simulink model "RobotCode_R2022b"  (R2022b)
settings: Solver=ode3  StartTime=0.0  StopTime=inf  RelTol=1e-3  EnableMultiTasking=on
undefined symbols (not defined in the file or in its folder): CPR, DRV_GAIN, GR, T
libraries: cstblocks x8, simulink x8, arduinosensorlib x5, dspsigops x1
settings Model: FPTRunName=Active  ExtModeTrigDuration=2  Creator=20181889  LastModifiedBy=Rafael
settings SolverCC: AlgebraicLoopSolver=TrustRegion  AutoInsertRateTranBlk=on
settings DataIOCC: LimitDataPoints=on  SaveFormat=Array
settings OptimizationCC: ReuseModelBlockBuffer=on  ExpressionDepthLimit=2147483647  LifeSpan=Inf  MaxStackSize=64
settings DebuggingCC: UnderspecifiedInitializationDetection=Classic  MergeDetectMultiDrivingBlocksExec=none  FcnCallInpInsideContextMsg=warning  UnconnectedInputMsg=warning  UnconnectedOutputMsg=warning  UnconnectedLineMsg=warning  AllowSymbolicDim=off  StateNameClashWarn=warning  SFUnexpectedBacktrackingDiag=warning  SFNoUnconditionalDefaultTransitionDiag=warning  SFExecutionAtInitializationDiag=none  ArithmeticOperatorsInVariantConditions=warning
settings HardwareCC: ProdBitPerPointer=32  ProdBitPerSizeT=32  ProdBitPerPtrDiffT=32  ProdLargestAtomicInteger=Long  ProdLargestAtomicFloat=Double  ProdWordSize=32  ProdHWDeviceType=ARM Compatible->ARM Cortex
settings ModelReferenceCC: EnableRefExpFcnMdlSchedulingChecks=on  PropagateSignalLabelsOutOfModel=off
settings SFSimCC: SimUseLocalCustomCode=off  CustomCodeUndefinedFunction=UseInterfaceOnly
settings RTWCC: Description=Embedded Coder  SystemTargetFile=ert.tlc  HardwareBoard=Arduino Due  TemplateMakefile=ert_default_tmf  GenerateReport=on  RTWVerbose=off  RTWUseLocalCustomCode=off  Toolchain=Arduino ARM  BuildConfiguration=Faster Runs  LaunchReport=on
settings CodeAppCC: ForceParamTrailComments=on  OperatorAnnotations=on  StateflowObjectComments=on  MATLABSourceComments=on
settings ERTTargetCC: TargetLangStandard=C99 (ISO)  MultiwordLength=2048  ERTCustomFileBanners=off  SupportContinuousTime=on  SupportNonInlinedSFcns=on  RemoveResetFunc=off  SupportVariableSizeSignals=on  ModelStepFunctionPrototypeControlCompliant=off  ExtModeTransport=3  ExtModeStaticAlloc=on  ExtModeStaticAllocSize=24576  ExtModeMexFile=ext_xcp  ExtModeIntrfLevel=Level2 - Open
settings ConfigComp: CovMetricSettings=dw  CovSaveCumulativeToWorkspaceVar=on  CovSaveSingleToWorkspaceVar=on  CovExternalEMLEnable=off  CovSFcnEnable=off

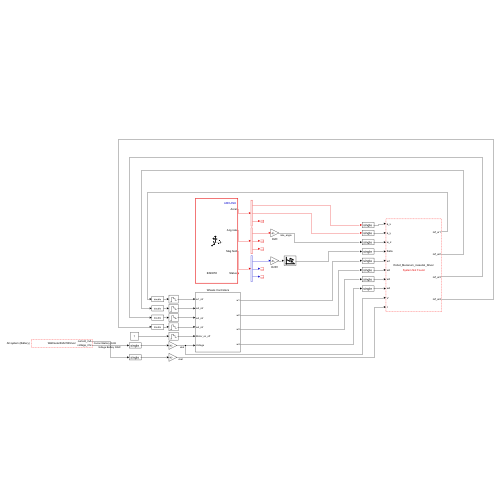
[thumbnail: Simulink's stored preview of the top-level diagram]
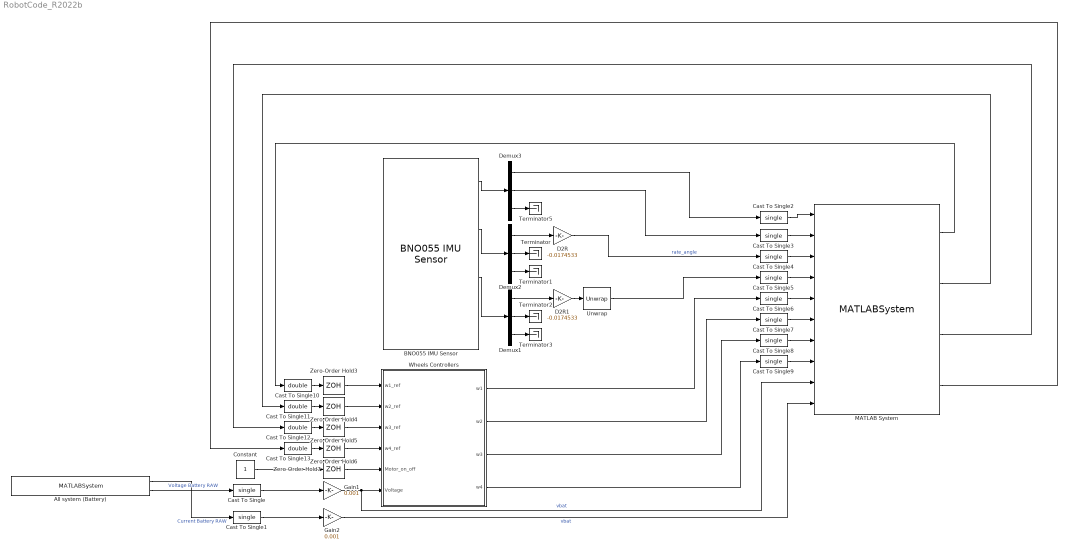
== system RobotCode_R2022b ==
  All system (Battery) : MATLABSystem  System=WattmeterINA219Driver  id=0  wire_number=0  address=45  SampleTime=T
      mask Type: WattmeterINA219Driver
      mask Display:
      | disp('WattmeterINA219Driver');
      | port_label('output',1,'current_mA');
      | port_label('output',2,'voltage_mV');
  BNO055 IMU Sensor : arduinosensorlib/BNO055 IMU Sensor  SlaveAddress=0x29  OperationMode=Fusion  Accel=on  AngularRate=on  MagField=off  EulerAngles=on  Quat=off  LinearAccel=off  GravityVector=off  Status=off  Timestamp=off  AccelRange=4G  AccelBW=62.5 Hz  GyroRange=2000 dps  GyroBW=32 Hz  MagODR=10 Hz  spf=1  SampleTime=T  blockPlatform=ARDUINO  QueueSizeFactor=1
  Cast To Single{,1..9} (10 alike) : DataTypeConversion  OutDataTypeStr=single  SaturateOnIntegerOverflow=off  RndMeth=Floor
  Cast To Single{10..13} (4 alike) : DataTypeConversion  OutDataTypeStr=double  SaturateOnIntegerOverflow=off  RndMeth=Floor
  Constant : Constant
  D2R : Gain  Gain=-0.0174533
  D2R1 : Gain  Gain=-0.0174533
  Demux1 : Demux  Outputs=3
  Demux2 : Demux  Outputs=3
  Demux3 : Demux  Outputs=3
  Gain1 : Gain  Gain=0.001
  Gain2 : Gain  Gain=0.001
  MATLAB System : MATLABSystem  System=Robot_Mecanum_rosserial_Driver  SampleTime=T
      mask Type: Robot_Mecanum_rosserial_Driver
      mask Display:
      | disp('Robot_Mecanum_rosserial_Driver');
      | port_label('input',1,'a_x');
      | port_label('input',2,'a_y');
      | port_label('input',3,'w_z');
      | port_label('input',4,'theta');
      | port_label('input',5,'w1');
      | port_label('input',6,'w2');
      | port_label('input',7,'w3');
      | port_label('input',8,'w4');
      | port_label('input',9,'V');
      | port_label('input',10,'I');
      | port_label('output',1,'ref_w1');
      | port_label('output',2,'ref_w2');
      | port_label('output',3,'ref_w3');
      | port_label('output',4,'ref_w4');
  Terminator{,1..3,5} (5 alike) : Terminator
  Unwrap : dspsigops/Unwrap  tol=pi  InputProcessing=Columns as channels (frame based)  running=off
  Wheels Controllers : Subsystem
  Zero-Order Hold{3..7} (5 alike) : ZeroOrderHold  SampleTime=T
  wires:
  All system (Battery)/2 -> Cast To Single/1  "Voltage Battery RAW"
  Cast To Single/1 -> Gain1/1
  Gain1/1 -> MATLAB System/9, Wheels Controllers/6(Voltage)  "vbat"
  Zero-Order Hold3/1 -> Wheels Controllers/1(w1_ref)
  Zero-Order Hold4/1 -> Wheels Controllers/2(w2_ref)
  Zero-Order Hold5/1 -> Wheels Controllers/3(w3_ref)
  Zero-Order Hold6/1 -> Wheels Controllers/4(w4_ref)
  Zero-Order Hold7/1 -> Wheels Controllers/5(Motor_on_off)
  Demux2/3 -> Terminator1/1
  BNO055 IMU Sensor/3 -> Demux1/1
  Demux2/2 -> Terminator/1
  Demux1/2 -> Terminator2/1
  BNO055 IMU Sensor/2 -> Demux2/1
  Demux1/3 -> Terminator3/1
  D2R1/1 -> Unwrap/1
  Demux2/1 -> D2R/1
  Demux1/1 -> D2R1/1
  All system (Battery)/1 -> Cast To Single1/1  "Current Battery RAW"
  Cast To Single1/1 -> Gain2/1
  Demux3/1 -> Cast To Single2/1
  Demux3/3 -> Terminator5/1
  Demux3/2 -> Cast To Single3/1
  BNO055 IMU Sensor/1 -> Demux3/1
  Cast To Single2/1 -> MATLAB System/1
  Cast To Single3/1 -> MATLAB System/2
  Cast To Single4/1 -> MATLAB System/3
  Cast To Single5/1 -> MATLAB System/4
  D2R/1 -> Cast To Single4/1  "rate_angle"
  Unwrap/1 -> Cast To Single5/1
  Wheels Controllers/1(w1) -> Cast To Single6/1
  Cast To Single6/1 -> MATLAB System/5
  Cast To Single7/1 -> MATLAB System/6
  Wheels Controllers/2(w2) -> Cast To Single7/1
  Cast To Single8/1 -> MATLAB System/7
  Wheels Controllers/3(w3) -> Cast To Single8/1
  Cast To Single9/1 -> MATLAB System/8
  Wheels Controllers/4(w4) -> Cast To Single9/1
  Gain2/1 -> MATLAB System/10  "vbat"
  MATLAB System/1 -> Cast To Single10/1
  MATLAB System/2 -> Cast To Single11/1
  MATLAB System/3 -> Cast To Single12/1
  MATLAB System/4 -> Cast To Single13/1
  Constant/1 -> Zero-Order Hold7/1
  Cast To Single10/1 -> Zero-Order Hold3/1
  Cast To Single11/1 -> Zero-Order Hold4/1
  Cast To Single12/1 -> Zero-Order Hold5/1
  Cast To Single13/1 -> Zero-Order Hold6/1

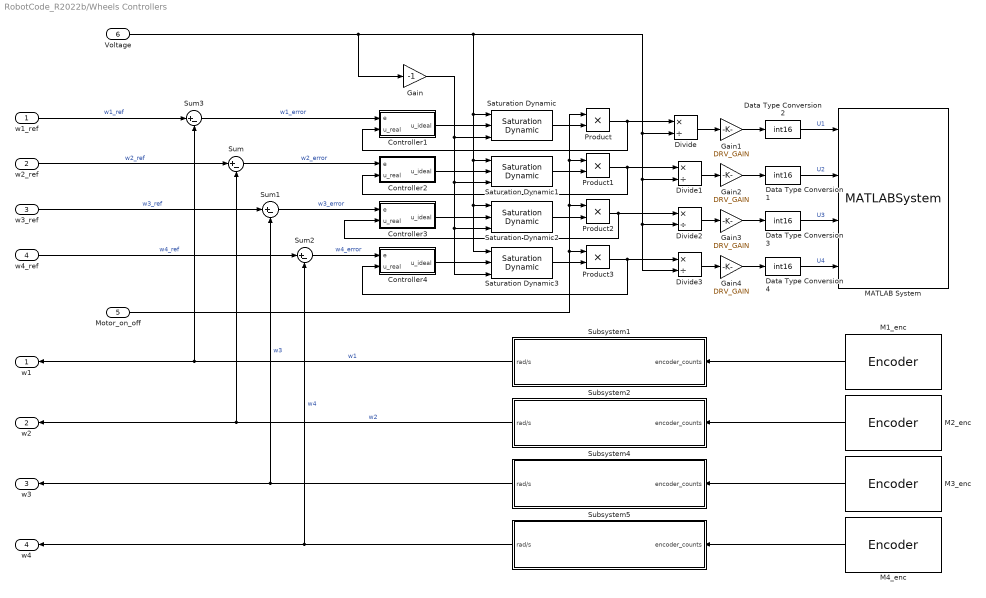
== system RobotCode_R2022b/Wheels Controllers ==
  w1_ref : Inport
  w2_ref : Inport  Port=2
  w3_ref : Inport  Port=3
  w4_ref : Inport  Port=4
  Motor_on_off : Inport  Port=5
  Voltage : Inport  Port=6
  Controller1 : Subsystem
  Controller2 : Subsystem
  Controller3 : Subsystem
  Controller4 : Subsystem
  Data Type Conversion{1..4} (4 alike) : DataTypeConversion  OutDataTypeStr=int16  SaturateOnIntegerOverflow=off  RndMeth=Floor
  Divide{,1..3} (4 alike) : Product  Inputs=*/
  Gain : Gain  Gain=-1
  Gain{1..4} (4 alike) : Gain  Gain=DRV_GAIN
  M1_enc : arduinosensorlib/Encoder  InputA=5  InputB=4  Mode=No reset  SampleTime=T
  M2_enc : arduinosensorlib/Encoder  InputA=3  InputB=2  Mode=No reset  SampleTime=T
  M3_enc : arduinosensorlib/Encoder  InputA=9  InputB=8  Mode=No reset  SampleTime=T
  M4_enc : arduinosensorlib/Encoder  InputA=7  InputB=6  Mode=No reset  SampleTime=T
  MATLAB System : MATLABSystem  System=AFMSV2Driver  SampleTime=T
      mask Type: AFMSV2Driver
      mask Display:
      | disp('AFMSV2Driver');
      | port_label('input',1,'U1');
      | port_label('input',2,'U2');
      | port_label('input',3,'U3');
      | port_label('input',4,'U4');
  Product{,1..3} (4 alike) : Product
  Saturation Dynamic{,1..3} (4 alike) : simulink/Discontinuities/Saturation Dynamic  OutMin=[]  OutMax=[]  OutDataTypeStr=Inherit: Same as second input  OutDataType=fixdt(1, 16)  OutScaling=2^-10  DoSatur=off
  Subsystem1 : Subsystem
  Subsystem2 : Subsystem
  Subsystem4 : Subsystem
  Subsystem5 : Subsystem
  Sum{,1..3} (4 alike) : Sum  Inputs=|+-
  w1 : Outport
  w2 : Outport  Port=2
  w3 : Outport  Port=3
  w4 : Outport  Port=4
  wires:
  M2_enc/1 -> Subsystem2/1(encoder_counts)
  Subsystem2/1(rad/s) -> w2/1, Sum/2  "w2"
  Subsystem4/1(rad/s) -> w3/1, Sum1/2  "w3"
  M3_enc/1 -> Subsystem4/1(encoder_counts)
  M1_enc/1 -> Subsystem1/1(encoder_counts)
  M4_enc/1 -> Subsystem5/1(encoder_counts)
  Subsystem5/1(rad/s) -> w4/1, Sum2/2  "w4"
  Subsystem1/1(rad/s) -> w1/1, Sum3/2  "w1"
  w2_ref/1 -> Sum/1  "w2_ref"
  Sum/1 -> Controller2/1(e)  "w2_error"
  w3_ref/1 -> Sum1/1  "w3_ref"
  Sum1/1 -> Controller3/1(e)  "w3_error"
  w4_ref/1 -> Sum2/1  "w4_ref"
  w1_ref/1 -> Sum3/1  "w1_ref"
  Sum2/1 -> Controller4/1(e)  "w4_error"
  Sum3/1 -> Controller1/1(e)  "w1_error"
  Controller1/1("u_ideal ") -> Saturation Dynamic/2
  Controller2/1("u_ideal ") -> Saturation Dynamic1/2
  Controller3/1("u_ideal ") -> Saturation Dynamic2/2
  Controller4/1("u_ideal ") -> Saturation Dynamic3/2
  Voltage/1 -> Gain/1, Saturation Dynamic3/1, Saturation Dynamic2/1, Saturation Dynamic1/1, Saturation Dynamic/1, Divide/2, Divide1/2, Divide2/2, Divide3/2
  Gain/1 -> Saturation Dynamic3/3, Saturation Dynamic2/3, Saturation Dynamic1/3, Saturation Dynamic/3
  Divide/1 -> Gain1/1
  Divide1/1 -> Gain2/1
  Divide2/1 -> Gain3/1
  Divide3/1 -> Gain4/1
  Data Type Conversion2/1 -> MATLAB System/1  "U1"
  Data Type Conversion1/1 -> MATLAB System/2  "U2"
  Data Type Conversion3/1 -> MATLAB System/3  "U3"
  Data Type Conversion4/1 -> MATLAB System/4  "U4"
  Product3/1 -> Controller4/2(u_real), Divide3/1
  Product1/1 -> Controller2/2(u_real), Divide1/1
  Product/1 -> Controller1/2(u_real), Divide/1
  Saturation Dynamic1/1 -> Product1/2
  Product2/1 -> Controller3/2(u_real), Divide2/1
  Motor_on_off/1 -> Product/1, Product1/1, Product2/1, Product3/1
  Saturation Dynamic/1 -> Product/2
  Saturation Dynamic2/1 -> Product2/2
  Saturation Dynamic3/1 -> Product3/2
  Gain3/1 -> Data Type Conversion3/1
  Gain4/1 -> Data Type Conversion4/1
  Gain2/1 -> Data Type Conversion1/1
  Gain1/1 -> Data Type Conversion2/1

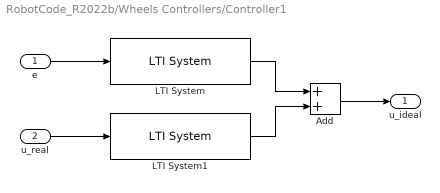
== system RobotCode_R2022b/Wheels Controllers/Controller1 ==
  e : Inport
  u_real : Inport  Port=2
  Add : Sum
  LTI System : cstblocks/LTI System  sys=M_tfEd  IC=[]
  LTI System1 : cstblocks/LTI System  sys=M_tfAd  IC=[]
  "u_ideal " : Outport
  wires:
  e/1 -> LTI System/1
  LTI System1/1 -> Add/2
  LTI System/1 -> Add/1
  Add/1 -> "u_ideal "/1
  u_real/1 -> LTI System1/1

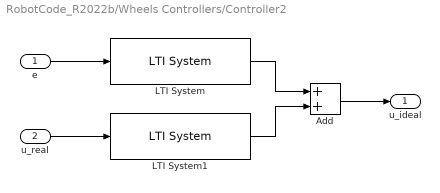
== system RobotCode_R2022b/Wheels Controllers/Controller2 ==
  e : Inport
  u_real : Inport  Port=2
  Add : Sum
  LTI System : cstblocks/LTI System  sys=M_tfEd  IC=[]
  LTI System1 : cstblocks/LTI System  sys=M_tfAd  IC=[]
  "u_ideal " : Outport
  wires:
  e/1 -> LTI System/1
  LTI System1/1 -> Add/2
  LTI System/1 -> Add/1
  Add/1 -> "u_ideal "/1
  u_real/1 -> LTI System1/1

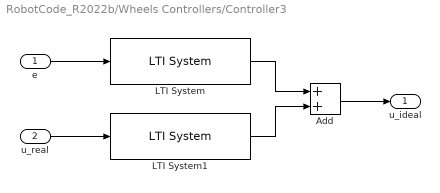
== system RobotCode_R2022b/Wheels Controllers/Controller3 ==
  e : Inport
  u_real : Inport  Port=2
  Add : Sum
  LTI System : cstblocks/LTI System  sys=M_tfEd  IC=[]
  LTI System1 : cstblocks/LTI System  sys=M_tfAd  IC=[]
  "u_ideal " : Outport
  wires:
  e/1 -> LTI System/1
  LTI System1/1 -> Add/2
  LTI System/1 -> Add/1
  Add/1 -> "u_ideal "/1
  u_real/1 -> LTI System1/1

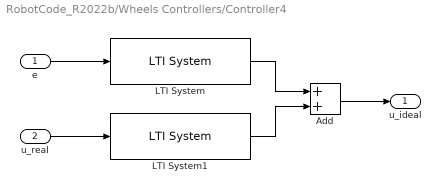
== system RobotCode_R2022b/Wheels Controllers/Controller4 ==
  e : Inport
  u_real : Inport  Port=2
  Add : Sum
  LTI System : cstblocks/LTI System  sys=M_tfEd  IC=[]
  LTI System1 : cstblocks/LTI System  sys=M_tfAd  IC=[]
  "u_ideal " : Outport
  wires:
  e/1 -> LTI System/1
  LTI System1/1 -> Add/2
  LTI System/1 -> Add/1
  Add/1 -> "u_ideal "/1
  u_real/1 -> LTI System1/1

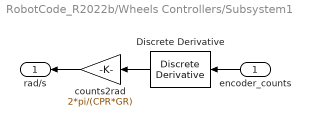
== system RobotCode_R2022b/Wheels Controllers/Subsystem1 ==
  encoder_counts : Inport
  Discrete Derivative : simulink/Discrete/Discrete Derivative  gainval=1.0  ICPrevScaledInput=0.0  OutMin=[]  OutMax=[]  OutDataType=fixdt(1, 16)  OutScaling=2^-10  DoSatur=off
  counts2rad : Gain  Gain=2*pi/(CPR*GR)
  rad/s : Outport
  wires:
  counts2rad/1 -> rad/s/1
  encoder_counts/1 -> Discrete Derivative/1
  Discrete Derivative/1 -> counts2rad/1

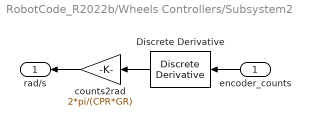
== system RobotCode_R2022b/Wheels Controllers/Subsystem2 ==
  encoder_counts : Inport
  Discrete Derivative : simulink/Discrete/Discrete Derivative  gainval=1.0  ICPrevScaledInput=0.0  OutMin=[]  OutMax=[]  OutDataType=fixdt(1, 16)  OutScaling=2^-10  DoSatur=off
  counts2rad : Gain  Gain=2*pi/(CPR*GR)
  rad/s : Outport
  wires:
  counts2rad/1 -> rad/s/1
  encoder_counts/1 -> Discrete Derivative/1
  Discrete Derivative/1 -> counts2rad/1

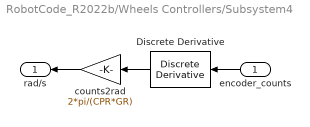
== system RobotCode_R2022b/Wheels Controllers/Subsystem4 ==
  encoder_counts : Inport
  Discrete Derivative : simulink/Discrete/Discrete Derivative  gainval=1.0  ICPrevScaledInput=0.0  OutMin=[]  OutMax=[]  OutDataType=fixdt(1, 16)  OutScaling=2^-10  DoSatur=off
  counts2rad : Gain  Gain=2*pi/(CPR*GR)
  rad/s : Outport
  wires:
  counts2rad/1 -> rad/s/1
  encoder_counts/1 -> Discrete Derivative/1
  Discrete Derivative/1 -> counts2rad/1

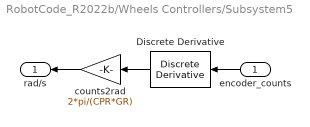
== system RobotCode_R2022b/Wheels Controllers/Subsystem5 ==
  encoder_counts : Inport
  Discrete Derivative : simulink/Discrete/Discrete Derivative  gainval=1.0  ICPrevScaledInput=0.0  OutMin=[]  OutMax=[]  OutDataType=fixdt(1, 16)  OutScaling=2^-10  DoSatur=off
  counts2rad : Gain  Gain=2*pi/(CPR*GR)
  rad/s : Outport
  wires:
  counts2rad/1 -> rad/s/1
  encoder_counts/1 -> Discrete Derivative/1
  Discrete Derivative/1 -> counts2rad/1
